simulink model "prob9"  (R2020b)
settings: Solver=VariableStepAuto  StartTime=0.0  StopTime=10.0  RelTol=1e-3
settings Model: Creator=AVM  LastModifiedBy=AVM

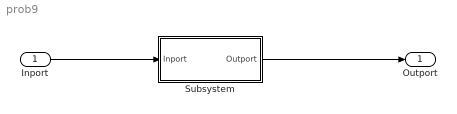
== system prob9 ==
  Inport : Inport
  Subsystem : Subsystem
  Outport : Outport
  wires:
  Inport/1 -> Subsystem/1(Inport)
  Subsystem/1(Outport) -> Outport/1

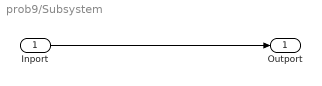
== system prob9/Subsystem ==
  Inport : Inport
  Outport : Outport
  wires:
  Inport/1 -> Outport/1
